simulink model "exercise_5_part_b"  (Simulink 7.1)
settings: Solver=ode1  StartTime=0.0  StopTime=10.0  FixedStep=T  RelTol=1e-3
undefined symbols (not defined in the file): I_half_of_the_act_Pitch, I_half_of_the_act_Roll, Ilink, Iload, Llink, Mact, Mlink, Mload, Ract, Rload, Wact
libraries: mblibv1 x31, simulink x3
settings Model: Creator=muinul  LastModifiedBy=muinul  ExtModeAutoUpdateStatusClock=off
settings SimMechanicsCC: VisOnUpdateDiagram=on  VisDuringSimulation=on

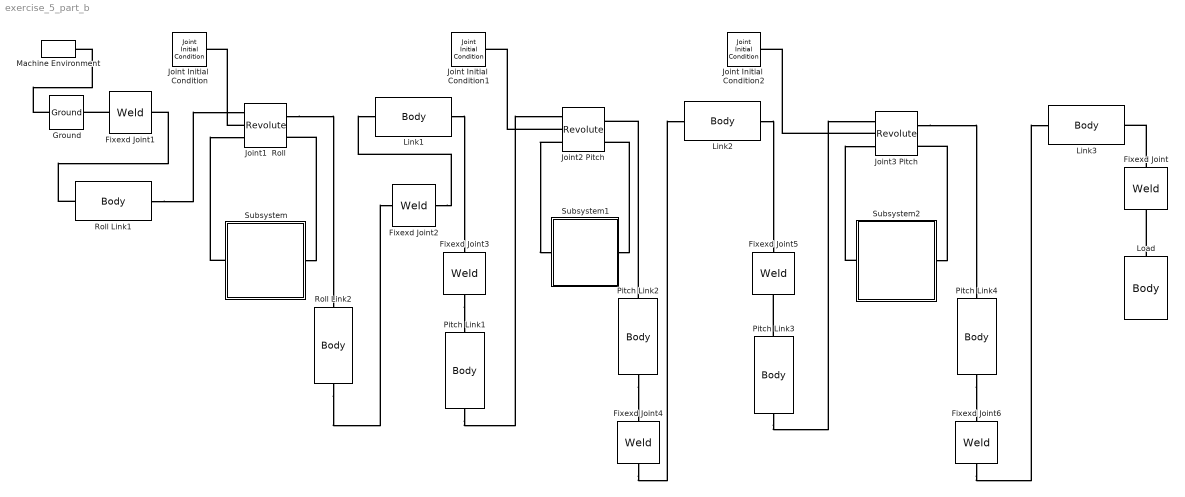
== system exercise_5_part_b ==
  Fixexd Joint{,3..6} (5 alike) : mblibv1/Joints/Weld  Orientation=down  DialogController=MECH.DynMechDlgSource  PhysicalDomain=mechanical  SubClassName=Unknown  LeftPortType=blob  RightPortType=blob  LConnTagsString=__newl0  RConnTagsString=__newr0  NumSAPorts=0  CutJoint=off  MarkAsCut=off  Primitives=weld  PrimitiveProps=W$WORLD$[0 0 0]$weld  DialogClass=JointBlock  WAxis=[0 0 0]
  Fixexd Joint1 : mblibv1/Joints/Weld  DialogController=MECH.DynMechDlgSource  PhysicalDomain=mechanical  SubClassName=Unknown  LeftPortType=blob  RightPortType=blob  LConnTagsString=__newl0  RConnTagsString=__newr0  NumSAPorts=0  CutJoint=off  MarkAsCut=off  Primitives=weld  PrimitiveProps=W$WORLD$[0 0 0]$weld  DialogClass=JointBlock  WAxis=[0 0 0]
  Fixexd Joint2 : mblibv1/Joints/Weld  DialogController=MECH.DynMechDlgSource  PhysicalDomain=mechanical  SubClassName=Unknown  LeftPortType=blob  RightPortType=blob  LConnTagsString=__newl0  RConnTagsString=__newr0  NumSAPorts=0  CutJoint=off  MarkAsCut=off  Primitives=weld  PrimitiveProps=W$WORLD$[0 0 0]$weld  DialogClass=JointBlock  WAxis=[0 0 0]
  Ground : mblibv1/Bodies/Ground  DialogController=MECH.DynMechDlgSource  SystemSampleTime=-1  LeftPortType=env  RightPortType=workingframe  PhysicalDomain=Mechanical  DialogClass=GroundBlock  CoordPosition=[0 Llink/2 0]  CoordPositionUnits=m  StateVectorMgrId=1  MachineId=[2 0]  ShowEnvPort=on
  Joint Initial  Condition : mblibv1/Sensors &  Actuators/Joint Initial Condition  DialogController=MECH.DynMechDlgSource  SystemSampleTime=-1  PhysicalDomain=mechanical  DialogClass=InitialConditionBlock  InitialConditions=P1$false$0$m$deg$0$m/s$deg/s#P2$false$0$m$deg$0$m/s$deg/s#P3$false$0$m$deg$0$m/s$deg/s#R1$false$0$m$deg$0$m/s$deg/s#R2$false$0$m$deg$0$m/s$deg/s#R3$false$0$m$deg$0$m/s$deg/s#S$false$0$m$deg$0$m/s$deg/s  P1PIC=0  P1VIC=0  P2PIC=0  P2VIC=0  P3PIC=0  P3VIC=0  R1PIC=0  R1VIC=0  R2PIC=0  R2VIC=0  R3PIC=0  R3VIC=0  SPIC=0  SVIC=0
  Joint Initial  Condition1 : mblibv1/Sensors &  Actuators/Joint Initial Condition  DialogController=MECH.DynMechDlgSource  SystemSampleTime=-1  PhysicalDomain=mechanical  DialogClass=InitialConditionBlock  InitialConditions=P1$false$0$m$deg$0$m/s$deg/s#P2$false$0$m$deg$0$m/s$deg/s#P3$false$0$m$deg$0$m/s$deg/s#R1$false$0$m$deg$0$m/s$deg/s#R2$false$0$m$deg$0$m/s$deg/s#R3$false$0$m$deg$0$m/s$deg/s#S$false$0$m$deg$0$m/s$deg/s  P1PIC=0  P1VIC=0  P2PIC=0  P2VIC=0  P3PIC=0  P3VIC=0  R1PIC=0  R1VIC=0  R2PIC=0  R2VIC=0  R3PIC=0  R3VIC=0  SPIC=0  SVIC=0
  Joint Initial  Condition2 : mblibv1/Sensors &  Actuators/Joint Initial Condition  DialogController=MECH.DynMechDlgSource  SystemSampleTime=-1  PhysicalDomain=mechanical  DialogClass=InitialConditionBlock  InitialConditions=P1$false$0$m$deg$0$m/s$deg/s#P2$false$0$m$deg$0$m/s$deg/s#P3$false$0$m$deg$0$m/s$deg/s#R1$false$0$m$deg$0$m/s$deg/s#R2$false$0$m$deg$0$m/s$deg/s#R3$false$0$m$deg$0$m/s$deg/s#S$false$0$m$deg$0$m/s$deg/s  P1PIC=0  P1VIC=0  P2PIC=0  P2VIC=0  P3PIC=0  P3VIC=0  R1PIC=0  R1VIC=0  R2PIC=0  R2VIC=0  R3PIC=0  R3VIC=0  SPIC=0  SVIC=0
  Joint1  Roll : mblibv1/Joints/Revolute  DialogController=MECH.DynMechDlgSource  PhysicalDomain=mechanical  SubClassName=Unknown  LeftPortType=blob  RightPortType=blob  LConnTagsString=__newl0|SA1|SA2  RConnTagsString=__newr0|SA1  NumSAPorts=3  CutJoint=off  MarkAsCut=off  Primitives=prismatic  PrimitiveProps=R1$World$[0 1 0]$revolute  DialogClass=JointBlock  R1Axis=[0 1 0]
  Joint2 Pitch : mblibv1/Joints/Revolute  DialogController=MECH.DynMechDlgSource  PhysicalDomain=mechanical  SubClassName=Unknown  LeftPortType=blob  RightPortType=blob  LConnTagsString=__newl0|SA1|SA2  RConnTagsString=__newr0|SA1  NumSAPorts=3  CutJoint=off  MarkAsCut=off  Primitives=prismatic  PrimitiveProps=R1$World$[0 0 1]$revolute  DialogClass=JointBlock  R1Axis=[0 0 1]
  Joint3 Pitch : mblibv1/Joints/Revolute  DialogController=MECH.DynMechDlgSource  PhysicalDomain=mechanical  SubClassName=Unknown  LeftPortType=blob  RightPortType=blob  LConnTagsString=__newl0|SA1|SA2  RConnTagsString=__newr0|SA1  NumSAPorts=3  CutJoint=off  MarkAsCut=off  Primitives=prismatic  PrimitiveProps=R1$World$[0 0 1]$revolute  DialogClass=JointBlock  R1Axis=[0 0 1]
  Link1 : mblibv1/Bodies/Body  DialogController=MECH.DynMechDlgSource  PhysicalDomain=mechanical  SubClassName=Unknown  LeftPortType=workingframe  RightPortType=workingframe  LConnTagsString=CS1  RConnTagsString=CS2  DialogClass=MechanicalBodyBlock  Mass=Mlink  MassUnits=kg  InertiaUnits=kg*m^2  Inertia=Ilink  Shape=Cylinder  ShapeDims=[1 1]  ShapeUnits=m  ShapeUse=false  Density=1  DensityUnits=kg/m^3  DensityUse=false  GraphicsMode=1  BodyColor=[0.5 0.5 0.5]  GraphicsObj=[]  AttachedToCS=1  CG=Left$CG$[0 Llink/2 0]$World$CS1$m$[0 0 0]$Euler X-Y-Z$deg$WORLD$false  WorkingFrames=Left$CS1$[0 0 0]$World$Adjoining$m$[0 0 0]$Euler X-Y-Z$deg$WORLD$true#Right$CS2$[0 Llink 0]$CG$CG$m$[0 0 0]$Euler X-Y-Z$deg$WORLD$true  CGPos=[0 Llink/2 0]  CGRot=[0 0 0]  CS0Pos=[]  CS0Rot=[]  CS1Pos=[0 0 0]  CS1Rot=[0 0 0]  CS2Pos=[0 Llink 0]  CS2Rot=[0 0 0]  CS3Pos=[]  CS3Rot=[]  CS4Pos=[]  CS4Rot=[]  CS5Pos=[]  CS5Rot=[]  CS6Pos=[]  CS6Rot=[]  CS7Pos=[]  CS7Rot=[]  CS8Pos=[]  CS8Rot=[]  CS9Pos=[]  CS9Rot=[]  CS10Pos=[]  CS10Rot=[]  CS11Pos=[]  CS11Rot=[]  CS12Pos=[]  CS12Rot=[]  CS13Pos=[]  CS13Rot=[]  CS14Pos=[]  CS14Rot=[]  CS15Pos=[]  CS15Rot=[]  CS16Pos=[]  CS16Rot=[]  CS17Pos=[]  CS17Rot=[]  CS18Pos=[]  CS18Rot=[]  CS19Pos=[]  CS19Rot=[]  CS20Pos=[]  CS20Rot=[]
  Link2 : mblibv1/Bodies/Body  DialogController=MECH.DynMechDlgSource  PhysicalDomain=mechanical  SubClassName=Unknown  LeftPortType=workingframe  RightPortType=workingframe  LConnTagsString=CS1  RConnTagsString=CS2  DialogClass=MechanicalBodyBlock  Mass=Mlink  MassUnits=kg  InertiaUnits=kg*m^2  Inertia=Ilink  Shape=Cylinder  ShapeDims=[1 1]  ShapeUnits=m  ShapeUse=false  Density=1  DensityUnits=kg/m^3  DensityUse=false  GraphicsMode=1  BodyColor=[0.5 0.5 0.5]  GraphicsObj=[]  AttachedToCS=1  CG=Left$CG$[0 Llink/2 0]$World$CS1$m$[0 0 0]$Euler X-Y-Z$deg$WORLD$false$none  WorkingFrames=Left$CS1$[0 0 0]$World$Adjoining$m$[0 0 0]$Euler X-Y-Z$deg$WORLD$true$none#Right$CS2$[0 Llink 0]$CG$CG$m$[0 0 0]$Euler X-Y-Z$deg$WORLD$true$none  CGPos=[0 Llink/2 0]  CGRot=[0 0 0]  CS0Pos=[]  CS0Rot=[]  CS1Pos=[0 0 0]  CS1Rot=[0 0 0]  CS2Pos=[0 Llink 0]  CS2Rot=[0 0 0]  CS3Pos=[]  CS3Rot=[]  CS4Pos=[]  CS4Rot=[]  CS5Pos=[]  CS5Rot=[]  CS6Pos=[]  CS6Rot=[]  CS7Pos=[]  CS7Rot=[]  CS8Pos=[]  CS8Rot=[]  CS9Pos=[]  CS9Rot=[]  CS10Pos=[]  CS10Rot=[]  CS11Pos=[]  CS11Rot=[]  CS12Pos=[]  CS12Rot=[]  CS13Pos=[]  CS13Rot=[]  CS14Pos=[]  CS14Rot=[]  CS15Pos=[]  CS15Rot=[]  CS16Pos=[]  CS16Rot=[]  CS17Pos=[]  CS17Rot=[]  CS18Pos=[]  CS18Rot=[]  CS19Pos=[]  CS19Rot=[]  CS20Pos=[]  CS20Rot=[]
  Link3 : mblibv1/Bodies/Body  DialogController=MECH.DynMechDlgSource  PhysicalDomain=mechanical  SubClassName=Unknown  LeftPortType=workingframe  RightPortType=workingframe  LConnTagsString=CS1  RConnTagsString=CS2  DialogClass=MechanicalBodyBlock  Mass=Mlink  MassUnits=kg  InertiaUnits=kg*m^2  Inertia=Ilink  Shape=Cylinder  ShapeDims=[1 1]  ShapeUnits=m  ShapeUse=false  Density=1  DensityUnits=kg/m^3  DensityUse=false  GraphicsMode=1  BodyColor=[0.5 0.5 0.5]  GraphicsObj=[]  AttachedToCS=1  CG=Left$CG$[0 Llink/2 0]$World$CS1$m$[0 0 0]$Euler X-Y-Z$deg$WORLD$false$none  WorkingFrames=Left$CS1$[0 0 0]$World$Adjoining$m$[0 0 0]$Euler X-Y-Z$deg$WORLD$true$none#Right$CS2$[0 Llink 0]$CG$CG$m$[0 0 0]$Euler X-Y-Z$deg$WORLD$true$none  CGPos=[0 Llink/2 0]  CGRot=[0 0 0]  CS0Pos=[]  CS0Rot=[]  CS1Pos=[0 0 0]  CS1Rot=[0 0 0]  CS2Pos=[0 Llink 0]  CS2Rot=[0 0 0]  CS3Pos=[]  CS3Rot=[]  CS4Pos=[]  CS4Rot=[]  CS5Pos=[]  CS5Rot=[]  CS6Pos=[]  CS6Rot=[]  CS7Pos=[]  CS7Rot=[]  CS8Pos=[]  CS8Rot=[]  CS9Pos=[]  CS9Rot=[]  CS10Pos=[]  CS10Rot=[]  CS11Pos=[]  CS11Rot=[]  CS12Pos=[]  CS12Rot=[]  CS13Pos=[]  CS13Rot=[]  CS14Pos=[]  CS14Rot=[]  CS15Pos=[]  CS15Rot=[]  CS16Pos=[]  CS16Rot=[]  CS17Pos=[]  CS17Rot=[]  CS18Pos=[]  CS18Rot=[]  CS19Pos=[]  CS19Rot=[]  CS20Pos=[]  CS20Rot=[]
  Load : mblibv1/Bodies/Body  Orientation=down  DialogController=MECH.DynMechDlgSource  PhysicalDomain=mechanical  SubClassName=Unknown  LeftPortType=workingframe  RightPortType=workingframe  LConnTagsString=CS1  RConnTagsString=CS2  DialogClass=MechanicalBodyBlock  Mass=Mload  MassUnits=kg  InertiaUnits=kg*m^2  Inertia=Iload  Shape=Cylinder  ShapeDims=[1 1]  ShapeUnits=m  ShapeUse=false  Density=1  DensityUnits=kg/m^3  DensityUse=false  GraphicsMode=1  BodyColor=[0.5 0.5 0.5]  GraphicsObj=[]  AttachedToCS=1  CG=Left$CG$[0 Rload 0]$World$CS1$m$[0 0 0]$Euler X-Y-Z$deg$WORLD$false$none  WorkingFrames=Left$CS1$[0 0 0]$World$Adjoining$m$[0 0 0]$Euler X-Y-Z$deg$WORLD$true$none#Right$CS2$[0 2*Rload 0]$World$CS1$m$[0 0 0]$Euler X-Y-Z$deg$WORLD$true$none  CGPos=[0 Rload 0]  CGRot=[0 0 0]  CS0Pos=[]  CS0Rot=[]  CS1Pos=[0 0 0]  CS1Rot=[0 0 0]  CS2Pos=[0 2*Rload 0]  CS2Rot=[0 0 0]  CS3Pos=[]  CS3Rot=[]  CS4Pos=[]  CS4Rot=[]  CS5Pos=[]  CS5Rot=[]  CS6Pos=[]  CS6Rot=[]  CS7Pos=[]  CS7Rot=[]  CS8Pos=[]  CS8Rot=[]  CS9Pos=[]  CS9Rot=[]  CS10Pos=[]  CS10Rot=[]  CS11Pos=[]  CS11Rot=[]  CS12Pos=[]  CS12Rot=[]  CS13Pos=[]  CS13Rot=[]  CS14Pos=[]  CS14Rot=[]  CS15Pos=[]  CS15Rot=[]  CS16Pos=[]  CS16Rot=[]  CS17Pos=[]  CS17Rot=[]  CS18Pos=[]  CS18Rot=[]  CS19Pos=[]  CS19Rot=[]  CS20Pos=[]  CS20Rot=[]
  Machine Environment : mblibv1/Bodies/Machine Environment  DialogController=MECH.DialogSource  SystemSampleTime=-1  PortType=env  PhysicalDomain=Mechanical  DialogTemplateClass=MECH.MachineEnvironment  SyncWhenCopied=off  Gravity=[0 -9.81 0]  GravityUnits=m/s^2  GravityAsSignal=off  Dimensionality=Auto-detect  AnalysisType=Inverse dynamics  LinearAssemblyTolerance=1e-3  LinearAssemblyToleranceUnits=m  AngularAssemblyTolerance=1e-3  AngularAssemblyToleranceUnits=rad  ConstraintSolverType=Stabilizing  ConstraintRelTolerance=1e-4  ConstraintAbsTolerance=1e-4  UseRobustSingularityHandling=off  RedundancyAnalysisToleranceType=Automatically select tolerance  RedundancyAnalysisTolerance=1e-14  StatePerturbationType=Fixed  PerturbationSize=1e-5  VisualizeMachine=on
  Pitch Link1 : mblibv1/Bodies/Body  Orientation=down  DialogController=MECH.DynMechDlgSource  PhysicalDomain=mechanical  SubClassName=Unknown  LeftPortType=workingframe  RightPortType=workingframe  LConnTagsString=CS1  RConnTagsString=CS2  DialogClass=MechanicalBodyBlock  Mass=Mact/2  MassUnits=kg  InertiaUnits=kg*m^2  Inertia=I_half_of_the_act_Pitch  Shape=Cylinder  ShapeDims=[1 1]  ShapeUnits=m  ShapeUse=false  Density=1  DensityUnits=kg/m^3  DensityUse=false  GraphicsMode=1  BodyColor=[0.5 0.5 0.5]  GraphicsObj=[]  AttachedToCS=1  CG=Left$CG$[0 Ract/2 0]$World$CS1$m$[0 0 0]$Euler X-Y-Z$deg$WORLD$false$none  WorkingFrames=Left$CS1$[0 0 0]$World$Adjoining$m$[0 0 0]$Euler X-Y-Z$deg$WORLD$true$none#Right$CS2$[0 Ract/2 -Wact/4]$World$CS1$m$[0 0 0]$Euler X-Y-Z$deg$WORLD$true$none  CGPos=[0 Ract/2 0]  CGRot=[0 0 0]  CS0Pos=[]  CS0Rot=[]  CS1Pos=[0 0 0]  CS1Rot=[0 0 0]  CS2Pos=[0 Ract/2 -Wact/4]  CS2Rot=[0 0 0]  CS3Pos=[]  CS3Rot=[]  CS4Pos=[]  CS4Rot=[]  CS5Pos=[]  CS5Rot=[]  CS6Pos=[]  CS6Rot=[]  CS7Pos=[]  CS7Rot=[]  CS8Pos=[]  CS8Rot=[]  CS9Pos=[]  CS9Rot=[]  CS10Pos=[]  CS10Rot=[]  CS11Pos=[]  CS11Rot=[]  CS12Pos=[]  CS12Rot=[]  CS13Pos=[]  CS13Rot=[]  CS14Pos=[]  CS14Rot=[]  CS15Pos=[]  CS15Rot=[]  CS16Pos=[]  CS16Rot=[]  CS17Pos=[]  CS17Rot=[]  CS18Pos=[]  CS18Rot=[]  CS19Pos=[]  CS19Rot=[]  CS20Pos=[]  CS20Rot=[]
  Pitch Link2 : mblibv1/Bodies/Body  Orientation=down  DialogController=MECH.DynMechDlgSource  PhysicalDomain=mechanical  SubClassName=Unknown  LeftPortType=workingframe  RightPortType=workingframe  LConnTagsString=CS1  RConnTagsString=CS2  DialogClass=MechanicalBodyBlock  Mass=Mact/2  MassUnits=kg  InertiaUnits=kg*m^2  Inertia=I_half_of_the_act_Pitch  Shape=Cylinder  ShapeDims=[1 1]  ShapeUnits=m  ShapeUse=false  Density=1  DensityUnits=kg/m^3  DensityUse=false  GraphicsMode=1  BodyColor=[0.5 0.5 0.5]  GraphicsObj=[]  AttachedToCS=1  CG=Left$CG$[0 0 -Wact/4]$World$CS1$m$[0 0 0]$Euler X-Y-Z$deg$WORLD$false$none  WorkingFrames=Left$CS1$[0 0 0]$World$Adjoining$m$[0 0 0]$Euler X-Y-Z$deg$WORLD$true$none#Right$CS2$[0 Ract/2 -Wact/4]$World$CS1$m$[0 0 0]$Euler X-Y-Z$deg$WORLD$true$none  CGPos=[0 0 -Wact/4]  CGRot=[0 0 0]  CS0Pos=[]  CS0Rot=[]  CS1Pos=[0 0 0]  CS1Rot=[0 0 0]  CS2Pos=[0 Ract/2 -Wact/4]  CS2Rot=[0 0 0]  CS3Pos=[]  CS3Rot=[]  CS4Pos=[]  CS4Rot=[]  CS5Pos=[]  CS5Rot=[]  CS6Pos=[]  CS6Rot=[]  CS7Pos=[]  CS7Rot=[]  CS8Pos=[]  CS8Rot=[]  CS9Pos=[]  CS9Rot=[]  CS10Pos=[]  CS10Rot=[]  CS11Pos=[]  CS11Rot=[]  CS12Pos=[]  CS12Rot=[]  CS13Pos=[]  CS13Rot=[]  CS14Pos=[]  CS14Rot=[]  CS15Pos=[]  CS15Rot=[]  CS16Pos=[]  CS16Rot=[]  CS17Pos=[]  CS17Rot=[]  CS18Pos=[]  CS18Rot=[]  CS19Pos=[]  CS19Rot=[]  CS20Pos=[]  CS20Rot=[]
  Pitch Link3 : mblibv1/Bodies/Body  Orientation=down  DialogController=MECH.DynMechDlgSource  PhysicalDomain=mechanical  SubClassName=Unknown  LeftPortType=workingframe  RightPortType=workingframe  LConnTagsString=CS1  RConnTagsString=CS2  DialogClass=MechanicalBodyBlock  Mass=Mact/2  MassUnits=kg  InertiaUnits=kg*m^2  Inertia=I_half_of_the_act_Pitch  Shape=Cylinder  ShapeDims=[1 1]  ShapeUnits=m  ShapeUse=false  Density=1  DensityUnits=kg/m^3  DensityUse=false  GraphicsMode=1  BodyColor=[0.5 0.5 0.5]  GraphicsObj=[]  AttachedToCS=1  CG=Left$CG$[0 Ract/2 0]$World$CS1$m$[0 0 0]$Euler X-Y-Z$deg$WORLD$false$none  WorkingFrames=Left$CS1$[0 0 0]$World$Adjoining$m$[0 0 0]$Euler X-Y-Z$deg$WORLD$true$none#Right$CS2$[0 Ract/2 -Wact/4]$World$CS1$m$[0 0 0]$Euler X-Y-Z$deg$WORLD$true$none  CGPos=[0 Ract/2 0]  CGRot=[0 0 0]  CS0Pos=[]  CS0Rot=[]  CS1Pos=[0 0 0]  CS1Rot=[0 0 0]  CS2Pos=[0 Ract/2 -Wact/4]  CS2Rot=[0 0 0]  CS3Pos=[]  CS3Rot=[]  CS4Pos=[]  CS4Rot=[]  CS5Pos=[]  CS5Rot=[]  CS6Pos=[]  CS6Rot=[]  CS7Pos=[]  CS7Rot=[]  CS8Pos=[]  CS8Rot=[]  CS9Pos=[]  CS9Rot=[]  CS10Pos=[]  CS10Rot=[]  CS11Pos=[]  CS11Rot=[]  CS12Pos=[]  CS12Rot=[]  CS13Pos=[]  CS13Rot=[]  CS14Pos=[]  CS14Rot=[]  CS15Pos=[]  CS15Rot=[]  CS16Pos=[]  CS16Rot=[]  CS17Pos=[]  CS17Rot=[]  CS18Pos=[]  CS18Rot=[]  CS19Pos=[]  CS19Rot=[]  CS20Pos=[]  CS20Rot=[]
  Pitch Link4 : mblibv1/Bodies/Body  Orientation=down  DialogController=MECH.DynMechDlgSource  PhysicalDomain=mechanical  SubClassName=Unknown  LeftPortType=workingframe  RightPortType=workingframe  LConnTagsString=CS1  RConnTagsString=CS2  DialogClass=MechanicalBodyBlock  Mass=Mact/2  MassUnits=kg  InertiaUnits=kg*m^2  Inertia=I_half_of_the_act_Pitch  Shape=Cylinder  ShapeDims=[1 1]  ShapeUnits=m  ShapeUse=false  Density=1  DensityUnits=kg/m^3  DensityUse=false  GraphicsMode=1  BodyColor=[0.5 0.5 0.5]  GraphicsObj=[]  AttachedToCS=1  CG=Left$CG$[0 0 -Wact/4]$World$CS1$m$[0 0 0]$Euler X-Y-Z$deg$WORLD$false$none  WorkingFrames=Left$CS1$[0 0 0]$World$Adjoining$m$[0 0 0]$Euler X-Y-Z$deg$WORLD$true$none#Right$CS2$[0 Ract/2 -Wact/4]$World$CS1$m$[0 0 0]$Euler X-Y-Z$deg$WORLD$true$none  CGPos=[0 0 -Wact/4]  CGRot=[0 0 0]  CS0Pos=[]  CS0Rot=[]  CS1Pos=[0 0 0]  CS1Rot=[0 0 0]  CS2Pos=[0 Ract/2 -Wact/4]  CS2Rot=[0 0 0]  CS3Pos=[]  CS3Rot=[]  CS4Pos=[]  CS4Rot=[]  CS5Pos=[]  CS5Rot=[]  CS6Pos=[]  CS6Rot=[]  CS7Pos=[]  CS7Rot=[]  CS8Pos=[]  CS8Rot=[]  CS9Pos=[]  CS9Rot=[]  CS10Pos=[]  CS10Rot=[]  CS11Pos=[]  CS11Rot=[]  CS12Pos=[]  CS12Rot=[]  CS13Pos=[]  CS13Rot=[]  CS14Pos=[]  CS14Rot=[]  CS15Pos=[]  CS15Rot=[]  CS16Pos=[]  CS16Rot=[]  CS17Pos=[]  CS17Rot=[]  CS18Pos=[]  CS18Rot=[]  CS19Pos=[]  CS19Rot=[]  CS20Pos=[]  CS20Rot=[]
  Roll Link1 : mblibv1/Bodies/Body  DialogController=MECH.DynMechDlgSource  PhysicalDomain=mechanical  SubClassName=Unknown  LeftPortType=workingframe  RightPortType=workingframe  LConnTagsString=CS1  RConnTagsString=CS2  DialogClass=MechanicalBodyBlock  Mass=Mact/2  MassUnits=kg  InertiaUnits=kg*m^2  Inertia=I_half_of_the_act_Roll  Shape=Cylinder  ShapeDims=[1 1]  ShapeUnits=m  ShapeUse=false  Density=1  DensityUnits=kg/m^3  DensityUse=false  GraphicsMode=1  BodyColor=[0.5 0.5 0.5]  GraphicsObj=[]  AttachedToCS=1  CG=Left$CG$[0 Wact/4 0]$World$CS1$m$[0 0 0]$Euler X-Y-Z$deg$WORLD$false$none  WorkingFrames=Left$CS1$[0 0 0]$World$Adjoining$m$[0 0 0]$Euler X-Y-Z$deg$WORLD$true$none#Right$CS2$[0 Wact/2 0]$CS1$CS1$m$[0 0 0]$Euler X-Y-Z$deg$WORLD$true$none  CGPos=[0 Wact/4 0]  CGRot=[0 0 0]  CS0Pos=[]  CS0Rot=[]  CS1Pos=[0 0 0]  CS1Rot=[0 0 0]  CS2Pos=[0 Wact/2 0]  CS2Rot=[0 0 0]  CS3Pos=[]  CS3Rot=[]  CS4Pos=[]  CS4Rot=[]  CS5Pos=[]  CS5Rot=[]  CS6Pos=[]  CS6Rot=[]  CS7Pos=[]  CS7Rot=[]  CS8Pos=[]  CS8Rot=[]  CS9Pos=[]  CS9Rot=[]  CS10Pos=[]  CS10Rot=[]  CS11Pos=[]  CS11Rot=[]  CS12Pos=[]  CS12Rot=[]  CS13Pos=[]  CS13Rot=[]  CS14Pos=[]  CS14Rot=[]  CS15Pos=[]  CS15Rot=[]  CS16Pos=[]  CS16Rot=[]  CS17Pos=[]  CS17Rot=[]  CS18Pos=[]  CS18Rot=[]  CS19Pos=[]  CS19Rot=[]  CS20Pos=[]  CS20Rot=[]
  Roll Link2 : mblibv1/Bodies/Body  Orientation=down  DialogController=MECH.DynMechDlgSource  PhysicalDomain=mechanical  SubClassName=Unknown  LeftPortType=workingframe  RightPortType=workingframe  LConnTagsString=CS1  RConnTagsString=CS2  DialogClass=MechanicalBodyBlock  Mass=Mact/2  MassUnits=kg  InertiaUnits=kg*m^2  Inertia=I_half_of_the_act_Roll  Shape=Cylinder  ShapeDims=[1 1]  ShapeUnits=m  ShapeUse=false  Density=1  DensityUnits=kg/m^3  DensityUse=false  GraphicsMode=1  BodyColor=[0.5 0.5 0.5]  GraphicsObj=[]  AttachedToCS=1  CG=Left$CG$[0 Wact/4 0]$World$CS1$m$[0 0 0]$Euler X-Y-Z$deg$WORLD$false$none  WorkingFrames=Left$CS1$[0 0 0]$World$Adjoining$m$[0 0 0]$Euler X-Y-Z$deg$WORLD$true$none#Right$CS2$[0 Wact/2 0]$CS1$CS1$m$[0 0 0]$Euler X-Y-Z$deg$WORLD$true$none  CGPos=[0 Wact/4 0]  CGRot=[0 0 0]  CS0Pos=[]  CS0Rot=[]  CS1Pos=[0 0 0]  CS1Rot=[0 0 0]  CS2Pos=[0 Wact/2 0]  CS2Rot=[0 0 0]  CS3Pos=[]  CS3Rot=[]  CS4Pos=[]  CS4Rot=[]  CS5Pos=[]  CS5Rot=[]  CS6Pos=[]  CS6Rot=[]  CS7Pos=[]  CS7Rot=[]  CS8Pos=[]  CS8Rot=[]  CS9Pos=[]  CS9Rot=[]  CS10Pos=[]  CS10Rot=[]  CS11Pos=[]  CS11Rot=[]  CS12Pos=[]  CS12Rot=[]  CS13Pos=[]  CS13Rot=[]  CS14Pos=[]  CS14Rot=[]  CS15Pos=[]  CS15Rot=[]  CS16Pos=[]  CS16Rot=[]  CS17Pos=[]  CS17Rot=[]  CS18Pos=[]  CS18Rot=[]  CS19Pos=[]  CS19Rot=[]  CS20Pos=[]  CS20Rot=[]
  Subsystem : Subsystem  Orientation=left
  Subsystem1 : Subsystem  Orientation=left
  Subsystem2 : Subsystem  Orientation=left
  connections:
  Fixexd Joint/LConn1 -- Link3/RConn1
  Load/LConn1 -- Fixexd Joint/RConn1
  Joint1  Roll/LConn2 -- Joint Initial  Condition/RConn1
  Joint2 Pitch/LConn2 -- Joint Initial  Condition1/RConn1
  Joint3 Pitch/LConn2 -- Joint Initial  Condition2/RConn1
  Subsystem1/LConn1 -- Joint2 Pitch/RConn2
  Joint2 Pitch/LConn3 -- Subsystem1/RConn1
  Subsystem2/LConn1 -- Joint3 Pitch/RConn2
  Subsystem2/RConn1 -- Joint3 Pitch/LConn3
  Subsystem/RConn1 -- Joint1  Roll/LConn3
  Ground/LConn1 -- Machine Environment/RConn1
  Fixexd Joint1/LConn1 -- Ground/RConn1
  Subsystem/LConn1 -- Joint1  Roll/RConn2
  Roll Link1/LConn1 -- Fixexd Joint1/RConn1
  Roll Link1/RConn1 -- Joint1  Roll/LConn1
  Joint1  Roll/RConn1 -- Roll Link2/LConn1
  Roll Link2/RConn1 -- Fixexd Joint2/LConn1
  Fixexd Joint2/RConn1 -- Link1/LConn1
  Link1/RConn1 -- Fixexd Joint3/LConn1
  Fixexd Joint3/RConn1 -- Pitch Link1/LConn1
  Pitch Link1/RConn1 -- Joint2 Pitch/LConn1
  Pitch Link2/LConn1 -- Joint2 Pitch/RConn1
  Pitch Link2/RConn1 -- Fixexd Joint4/LConn1
  Fixexd Joint4/RConn1 -- Link2/LConn1
  Link2/RConn1 -- Fixexd Joint5/LConn1
  Pitch Link3/LConn1 -- Fixexd Joint5/RConn1
  Pitch Link3/RConn1 -- Joint3 Pitch/LConn1
  Joint3 Pitch/RConn1 -- Pitch Link4/LConn1
  Pitch Link4/RConn1 -- Fixexd Joint6/LConn1
  Fixexd Joint6/RConn1 -- Link3/LConn1

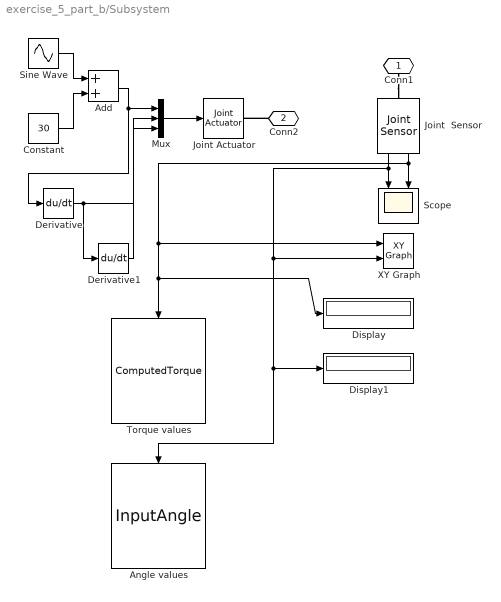
== system exercise_5_part_b/Subsystem ==
  Add : Sum  OutDataType=sfix(16)  OutScaling=2^-10
  Angle values : ToWorkspace  VariableName=InputAngle  SampleTime=-1  SaveFormat=Structure With Time
      settings: Orientation=down
  Constant : Constant  Value=30  OutDataType=sfix(16)  OutScaling=2^0
  Derivative : Derivative
  Derivative1 : Derivative
  Display : Display
  Display1 : Display
  Joint  Sensor : mblibv1/Sensors &  Actuators/Joint Sensor  Orientation=down  DialogController=MECH.DynMechDlgSource  SystemSampleTime=-1  PhysicalDomain=Mechanical  PortType=blob  Muxed=off  Pose=off  Angle=on  AngleUnits=deg  ArcVelocity=off  ArcVelocityUnits=deg/s  ArcAcceleration=off  ArcAccelerationUnits=deg/s^2  CoordPosition=on  CoordPositionUnits=m  Velocity=off  VelocityUnits=m/s  Acceleration=off  AccelerationUnits=m/s^2  Quaternion=on  QuaternionDT=off  QuaternionDDT=off  QuaternionUnits=off  OutputVector=[1]  ActiveIO=on  Width=2  DialogClass=MechanicalSensorBlock  Primitive=R1  Force=off  ForceUnits=N  Torque=on  TorqueUnits=N*m  ReferenceFrame=Absolute (World)  ReactionSensedSide=Base  ReactionReferenceFrame=Absolute (World)  ReactionForce=off  ReactionForceUnits=N  ReactionMoment=off  ReactionMomentUnits=N*m
  Joint Actuator : mblibv1/Sensors &  Actuators/Joint Actuator  DialogController=MECH.DynMechDlgSource  SystemSampleTime=-1  PhysicalDomain=Mechanical  PortType=blob  ActuationStyle=Motion  AngleUnits=deg  ArcVelocityUnits=deg/s  ArcAccelerationUnits=deg/s^2  CoordPositionUnits=m  VelocityUnits=m/s  AccelerationUnits=m/s^2  ForceUnits=N  TorqueUnits=N*m  ActiveIO=on  Width=3  DialogClass=MechanicalActuatorBlock  Primitive=R1  ReferenceFrame=Absolute (World)
  Mux : Mux  Inputs=3
  Scope : Scope  NumInputPorts=2
      settings: Orientation=down  YMin=-5~-5  YMax=5~5
  Sine Wave : Sin  Amplitude=30  Phase=-90*pi/180  SampleTime=0
  Torque values : ToWorkspace  VariableName=ComputedTorque  SampleTime=-1  SaveFormat=Structure With Time
      settings: Orientation=down
  XY Graph : simulink/Sinks/XY Graph  SystemSampleTime=-1  xmin=-1  xmax=1  ymin=-1  ymax=1  st=-1
  Conn1 : PMIOPort  Orientation=down  Port=1  Side=Left
  Conn2 : PMIOPort  Orientation=left  Port=2  Side=Right
  wires:
  Derivative/1 -> Mux/2, Derivative1/1
  Mux/1 -> Joint Actuator/1
  Derivative1/1 -> Mux/3
  Joint  Sensor/1 -> Scope/1, XY Graph/2, Angle values/1, Display1/1
  Joint  Sensor/2 -> Scope/2, XY Graph/1, Display/1, Torque values/1
  Add/1 -> Mux/1, Derivative/1
  Sine Wave/1 -> Add/1
  Constant/1 -> Add/2
  connections:
  Conn1/RConn1 -- Joint  Sensor/LConn1
  Conn2/RConn1 -- Joint Actuator/RConn1

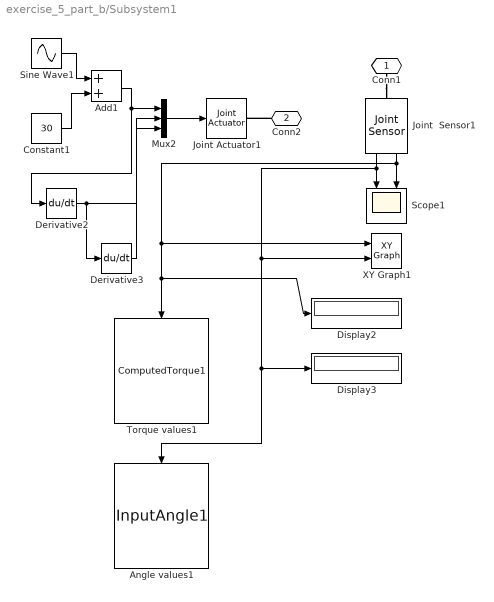
== system exercise_5_part_b/Subsystem1 ==
  Add1 : Sum  OutDataType=sfix(16)  OutScaling=2^-10
  Angle values1 : ToWorkspace  VariableName=InputAngle1  SampleTime=-1  SaveFormat=Structure With Time
      settings: Orientation=down
  Constant1 : Constant  Value=30  OutDataType=sfix(16)  OutScaling=2^0
  Derivative2 : Derivative
  Derivative3 : Derivative
  Display2 : Display
  Display3 : Display
  Joint  Sensor1 : mblibv1/Sensors &  Actuators/Joint Sensor  Orientation=down  DialogController=MECH.DynMechDlgSource  SystemSampleTime=-1  PhysicalDomain=Mechanical  PortType=blob  Muxed=off  Pose=off  Angle=on  AngleUnits=deg  ArcVelocity=off  ArcVelocityUnits=deg/s  ArcAcceleration=off  ArcAccelerationUnits=deg/s^2  CoordPosition=on  CoordPositionUnits=m  Velocity=off  VelocityUnits=m/s  Acceleration=off  AccelerationUnits=m/s^2  Quaternion=on  QuaternionDT=off  QuaternionDDT=off  QuaternionUnits=off  OutputVector=[1]  ActiveIO=on  Width=2  DialogClass=MechanicalSensorBlock  Primitive=R1  Force=off  ForceUnits=N  Torque=on  TorqueUnits=N*m  ReferenceFrame=Absolute (World)  ReactionSensedSide=Base  ReactionReferenceFrame=Absolute (World)  ReactionForce=off  ReactionForceUnits=N  ReactionMoment=off  ReactionMomentUnits=N*m
  Joint Actuator1 : mblibv1/Sensors &  Actuators/Joint Actuator  DialogController=MECH.DynMechDlgSource  SystemSampleTime=-1  PhysicalDomain=Mechanical  PortType=blob  ActuationStyle=Motion  AngleUnits=deg  ArcVelocityUnits=deg/s  ArcAccelerationUnits=deg/s^2  CoordPositionUnits=m  VelocityUnits=m/s  AccelerationUnits=m/s^2  ForceUnits=N  TorqueUnits=N*m  ActiveIO=on  Width=3  DialogClass=MechanicalActuatorBlock  Primitive=R1  ReferenceFrame=Absolute (World)
  Mux2 : Mux  Inputs=3
  Scope1 : Scope  NumInputPorts=2
      settings: Orientation=down  YMin=-5~-5  YMax=5~5
  Sine Wave1 : Sin  Amplitude=30  Phase=-90*pi/180  SampleTime=0
  Torque values1 : ToWorkspace  VariableName=ComputedTorque1  SampleTime=-1  SaveFormat=Structure With Time
      settings: Orientation=down
  XY Graph1 : simulink/Sinks/XY Graph  SystemSampleTime=-1  xmin=-1  xmax=1  ymin=-1  ymax=1  st=-1
  Conn1 : PMIOPort  Orientation=down  Port=1  Side=Left
  Conn2 : PMIOPort  Orientation=left  Port=2  Side=Right
  wires:
  Derivative2/1 -> Mux2/2, Derivative3/1
  Mux2/1 -> Joint Actuator1/1
  Derivative3/1 -> Mux2/3
  Joint  Sensor1/1 -> Scope1/1, XY Graph1/2, Angle values1/1, Display3/1
  Joint  Sensor1/2 -> Scope1/2, XY Graph1/1, Display2/1, Torque values1/1
  Add1/1 -> Mux2/1, Derivative2/1
  Constant1/1 -> Add1/2
  Sine Wave1/1 -> Add1/1
  connections:
  Conn1/RConn1 -- Joint  Sensor1/LConn1
  Conn2/RConn1 -- Joint Actuator1/RConn1

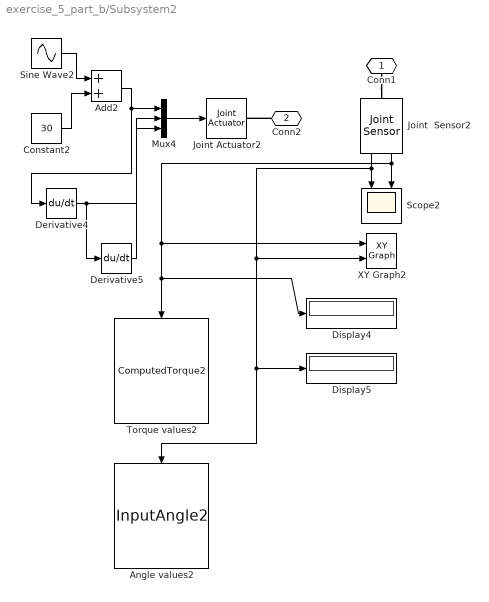
== system exercise_5_part_b/Subsystem2 ==
  Add2 : Sum  OutDataType=sfix(16)  OutScaling=2^-10
  Angle values2 : ToWorkspace  VariableName=InputAngle2  SampleTime=-1  SaveFormat=Structure With Time
      settings: Orientation=down
  Constant2 : Constant  Value=30  OutDataType=sfix(16)  OutScaling=2^0
  Derivative4 : Derivative
  Derivative5 : Derivative
  Display4 : Display
  Display5 : Display
  Joint  Sensor2 : mblibv1/Sensors &  Actuators/Joint Sensor  Orientation=down  DialogController=MECH.DynMechDlgSource  SystemSampleTime=-1  PhysicalDomain=Mechanical  PortType=blob  Muxed=off  Pose=off  Angle=on  AngleUnits=deg  ArcVelocity=off  ArcVelocityUnits=deg/s  ArcAcceleration=off  ArcAccelerationUnits=deg/s^2  CoordPosition=on  CoordPositionUnits=m  Velocity=off  VelocityUnits=m/s  Acceleration=off  AccelerationUnits=m/s^2  Quaternion=on  QuaternionDT=off  QuaternionDDT=off  QuaternionUnits=off  OutputVector=[1]  ActiveIO=on  Width=2  DialogClass=MechanicalSensorBlock  Primitive=R1  Force=off  ForceUnits=N  Torque=on  TorqueUnits=N*m  ReferenceFrame=Absolute (World)  ReactionSensedSide=Base  ReactionReferenceFrame=Absolute (World)  ReactionForce=off  ReactionForceUnits=N  ReactionMoment=off  ReactionMomentUnits=N*m
  Joint Actuator2 : mblibv1/Sensors &  Actuators/Joint Actuator  DialogController=MECH.DynMechDlgSource  SystemSampleTime=-1  PhysicalDomain=Mechanical  PortType=blob  ActuationStyle=Motion  AngleUnits=deg  ArcVelocityUnits=deg/s  ArcAccelerationUnits=deg/s^2  CoordPositionUnits=m  VelocityUnits=m/s  AccelerationUnits=m/s^2  ForceUnits=N  TorqueUnits=N*m  ActiveIO=on  Width=3  DialogClass=MechanicalActuatorBlock  Primitive=R1  ReferenceFrame=Absolute (World)
  Mux4 : Mux  Inputs=3
  Scope2 : Scope  NumInputPorts=2
      settings: Orientation=down  YMin=-5~-5  YMax=5~5  SaveName=ScopeData2
  Sine Wave2 : Sin  Amplitude=30  Phase=-90*pi/180  SampleTime=0
  Torque values2 : ToWorkspace  VariableName=ComputedTorque2  SampleTime=-1  SaveFormat=Structure With Time
      settings: Orientation=down
  XY Graph2 : simulink/Sinks/XY Graph  SystemSampleTime=-1  xmin=-1  xmax=1  ymin=-1  ymax=1  st=-1
  Conn1 : PMIOPort  Orientation=down  Port=1  Side=Left
  Conn2 : PMIOPort  Orientation=left  Port=2  Side=Right
  wires:
  Add2/1 -> Mux4/1, Derivative4/1
  Derivative4/1 -> Mux4/2, Derivative5/1
  Mux4/1 -> Joint Actuator2/1
  Derivative5/1 -> Mux4/3
  Joint  Sensor2/1 -> Scope2/1, XY Graph2/2, Angle values2/1, Display5/1
  Joint  Sensor2/2 -> Scope2/2, XY Graph2/1, Display4/1, Torque values2/1
  Constant2/1 -> Add2/2
  Sine Wave2/1 -> Add2/1
  connections:
  Conn1/RConn1 -- Joint  Sensor2/LConn1
  Conn2/RConn1 -- Joint Actuator2/RConn1
